simulink model "TEMPERATURESENSOR"  (R2023b)
settings: Solver=VariableStepAuto  StartTime=0.0  StopTime=10.0  RelTol=1e-3
settings Model: Creator=lucaerviati  LastModifiedBy=monis
settings DataIOCC: SaveOutput=off  SaveTime=off
settings OptimizationCC: ReuseModelBlockBuffer=off
settings GRTTargetCC: CombineOutputUpdateFcns=off  MatFileLogging=off

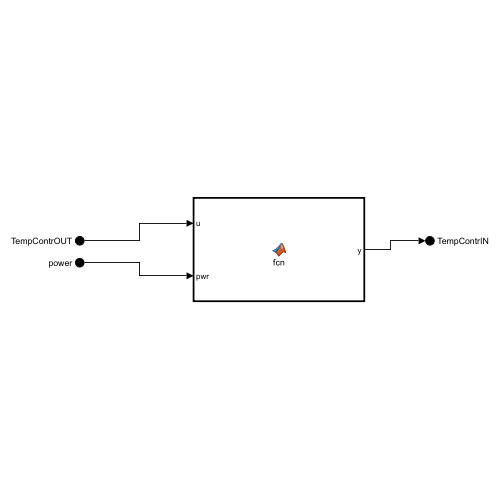
[thumbnail: Simulink's stored preview of the top-level diagram]
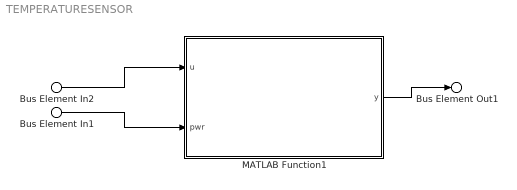
== system TEMPERATURESENSOR ==
  Bus Element In2 : Inport  PortName=TempContrOUT
  Bus Element In1 : Inport  Port=2  PortName=power
  MATLAB Function1 : MATLAB Function  TreatAsAtomicUnit=on
  Bus Element Out1 : Outport  PortName=TempContrIN
  wires:
  Bus Element In2/1 -> MATLAB Function1/1(u)
  Bus Element In1/1 -> MATLAB Function1/2(pwr)
  MATLAB Function1/1(y) -> Bus Element Out1/1

== matlab function TEMPERATURESENSOR/MATLAB Function1 ==
  data: u input; y output; pwr input
function y = fcn(u, pwr)

u = u*pwr;




y = u;
